simulink model "Model_FC_v14_Edit_for_Full_Scale_Fuel_Cell_GAS"  (R2017a)
settings: Solver=VariableStepAuto  StartTime=0  StopTime=10  FixedStep=0.01  MaxStep=1e-4  RelTol=1e-3  EnableMultiTasking=on
undefined symbols (not defined in the file): sigbuilder_block
libraries: powerlib x9, simulink x7, fl_lib x5, nesl_utility x3, powerlib_meascontrol x1
(part 1 of 3)
settings Model: SimulationMode=accelerator  Creator=Mina  LastModifiedBy=Mina
settings DataIOCC: LimitDataPoints=on  SaveFormat=Array
settings OptimizationCC: BlockReduction=off  ConditionallyExecuteInputs=off  LifeSpan=inf  SimCompilerOptimization=on  AccelVerboseBuild=on
settings DebuggingCC: SFUnexpectedBacktrackingDiag=warning  SFNoUnconditionalDefaultTransitionDiag=warning  SFExecutionAtInitializationDiag=none
settings HardwareCC: ProdBitPerPointer=32  ProdBitPerSizeT=32  ProdBitPerPtrDiffT=32  ProdLargestAtomicFloat=None  ProdIntDivRoundTo=Undefined  ProdEndianess=Unspecified  ProdWordSize=32  ProdHWDeviceType=32-bit Generic
settings ModelReferenceCC: PropagateSignalLabelsOutOfModel=off
settings GRTTargetCC: TargetLangStandard=C89/C90 (ANSI)  GeneratePreprocessorConditionals=Disable all
settings ConfigComp: CovMetricSettings=dw  CovHtmlReporting=on  CovSaveCumulativeToWorkspaceVar=on  CovSaveSingleToWorkspaceVar=on  CovExternalEMLEnable=off

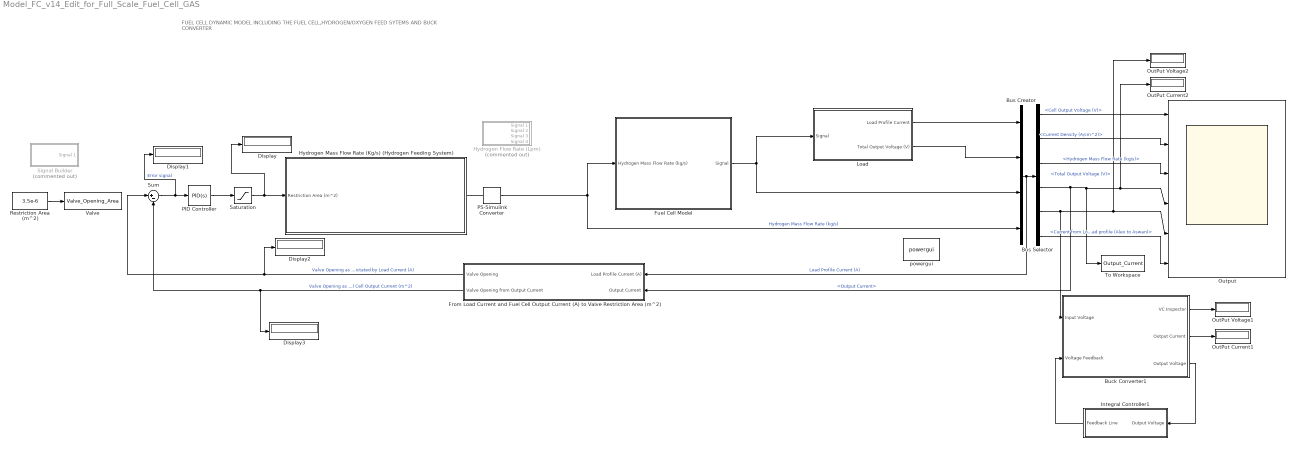
== system Model_FC_v14_Edit_for_Full_Scale_Fuel_Cell_GAS ==
  note: FUEL CELL DYNAMIC MODEL INCLUDING THE FUEL CELL,HYDROGEN/OXYGEN FEED SYTEMS AND BUCK CONVERTER
  Buck Converter1 : Subsystem
  Bus Creator : BusCreator  Inputs=4
  Bus Selector : BusSelector  OutputSignals=signal3.Cell Output Voltage (V),signal3.Current Density (A/cm^2),Hydrogen Mass Flow Rate (kg/s),signal3.Output Current,Total Output Voltage (V),Current from Load profile (Alex to Aswan)
  Display{,1..3} (4 alike) : Display
      Display settings: Decimation=100
  From Load Current and Fuel Cell Output Current (A) to Valve Restriction Area (m^2) : Subsystem
  Fuel Cell Model : Subsystem  mask(Fuel Cell Model){Temperature_c=80, Hydrogen_Pressure_atm=8, Air_Pressure_atm=8, Number_of_cells=235, Cell_Area_cm_squared=43.9714, Alpha_charge_Transfer_Coefficient=0.5, Exchange_Current_Density_i0=0.00000012246, Internal_Resistance_r=0.019, Amplification_Constant_Alpha1=0.085, Limiting_Current_Density_i_l=2, Mass_Transport_Limit_k=1.1, Dynamic_Response=[5 1]}
      mask prompts: Temperature_c "Temperature (c)"; Hydrogen_Pressure_atm "Hydrogen Pressure (atm)"; Air_Pressure_atm "Air Pressure (atm)"; Number_of_cells "Number Of Cells"; Cell_Area_cm_squared "Cell Area (cm^2)"; Alpha_charge_Transfer_Coefficient "Alpha (Charge Transfer Coefficient)"; Exchange_Current_Density_i0 "Exchange Current Density (i_0)(A/cm^2)"; Internal_Resistance_r "Internal Resistance (r)(Ohm)"; Amplification_Constant_Alpha1 "Amplification Constant (Alpha1)"; Limiting_Current_Density_i_l "Limiting Current Density (i_L)(A/cm^2)"; Mass_Transport_Limit_k "Mass Transport Limit (k)"; Dynamic_Response "Cell Dynamic Response (s)"
      mask help:
      | This is a mathematical Fuel Cell dynamic model. It operates under the Following Assumptions:
      | 1-The model is dynamic ,ie, it models the fuel cell behavior with respect to time.
      | 2-Fuel Cell Temperature is Constant.
      | 3-No Excess Hydrogen ,ie, Every Hydrogen molecule that enters the fuel cell Stack reacts to produce electricity.
      | 4-No excess Air.
      | 5-Concentration Losses are not calculated in the Model as we will never approach this region during operation.
      mask TypeOptions Temperature_c:
      | Stack Temperature
      | (C)/Value
      mask TypeOptions Hydrogen_Pressure_atm: Hydrogen Pressure (atm)/Value
      mask TypeOptions Air_Pressure_atm: Air Pressue (atm)/Value
      mask TypeOptions Number_of_cells: Number of Cells/Value
      mask TypeOptions Cell_Area_cm_squared:
      | Cell Area
      | (cm^2)/Value
      mask TypeOptions Alpha_charge_Transfer_Coefficient:
      | From Current Density (A//cm^2)
      | To
      | Overvoltages (V)/Activation Overvoltage/Alpha
      | Charge Transfer Coefficient1/Value
      mask TypeOptions Exchange_Current_Density_i0:
      | From Current Density (A//cm^2)
      | To
      | Overvoltages (V)/Activation Overvoltage/Reference Exchange Current Density
      | (I_0)1/Value
      mask TypeOptions Internal_Resistance_r:
      | From Current Density (A//cm^2)
      | To
      | Overvoltages (V)/Ohmic Overvoltage/Internal Resistance
      | (r)/Value
      mask TypeOptions Amplification_Constant_Alpha1:
      | From Current Density (A//cm^2)
      | To
      | Overvoltages (V)/Concentration Overvoltage/Amplification Constant
      | Alpha2/Value
      mask TypeOptions Limiting_Current_Density_i_l:
      | From Current Density (A//cm^2)
      | To
      | Overvoltages (V)/Concentration Overvoltage/Limiting Current
      | (i_L)1/Value
      mask TypeOptions Mass_Transport_Limit_k:
      | From Current Density (A//cm^2)
      | To
      | Overvoltages (V)/Concentration Overvoltage/Mass Transport Constant
      | (K)1/Value
      mask TypeOptions Dynamic_Response: Cell dynamic/Denominator
      mask Display: image(imread('power_fuelcell.png'));port_label('output',1,'m');
  Hydrogen Flow Rate (Lpm) : Subsystem  Tag=STV Subsys  Commented=on  LoadFcn=sigbuilder_block('load');  StartFcn=sigbuilder_block('start');  StopFcn=sigbuilder_block('stop');  ClipboardFcn=sigbuilder_block('clipboard');  mask(Sigbuilder block){tuvar=[0:10]}
      mask help: Simulink:masks:SigbuilderBlock_MD
      mask init:
      | if ~strcmp(get_param(bdroot(gcbh),'SimulationStatus'),'stopped') tuvar = sigbuilder_block('maskInit'); end
      settings: CopyFcn=sigbuilder_block('copy');  DeleteFcn=sigbuilder_block('delete');  ModelCloseFcn=sigbuilder_block('modelClose');  PreSaveFcn=sigbuilder_block('preSave');  PauseFcn=sigbuilder_block('pause');  ContinueFcn=sigbuilder_block('continue');  NameChangeFcn=sigbuilder_block('namechange');  OpenFcn=sigbuilder_block('open',[437.6 199.2 550.4 400 ]);  CloseFcn=sigbuilder_block('close');
      mask Display: plot(0, 0, 100, 100,[2, 2, 32, 32, 2], [68, 8, 8, 68, 68],[32, 2], [38, 38], [32, 19, 2],[53, 60, 44], [32, 17, 17, 2],[16, 16, 31, 31]);txt = getActiveGroup(gcbh);text(2, 100, txt,'verticalAlignment', 'top');
  Hydrogen Mass Flow Rate (Kg/s) (Hydrogen Feeding System) : Subsystem
  Integral Controller1 : Subsystem
  Load : Subsystem
  OutPut Current1 : Display
  OutPut Current2 : Display
  OutPut Voltage1 : Display
  OutPut Voltage2 : Display
  "Output " : Scope  NumInputPorts=6
  PID Controller : simulink/Continuous/PID Controller  Controller=PID  TimeDomain=Continuous-time  SampleTime=-1  IntegratorMethod=Forward Euler  FilterMethod=Forward Euler  Form=Parallel  UseFilter=on  ControllerParametersSource=internal  P=0.5  I=0.7  D=0.01  N=100  InitialConditionSource=internal  InitialConditionForIntegrator=0  InitialConditionForFilter=0  ExternalReset=none  LimitOutput=on  UpperSaturationLimit=1.5e-5  LowerSaturationLimit=-inf  LinearizeAsGain=on  AntiWindupMode=none  Kb=1  TrackingMode=off  Kt=1  PParamMin=[]  PParamMax=[]  IParamMin=[]  IParamMax=[]  DParamMin=[]  DParamMax=[]  NParamMin=[]  NParamMax=[]  KbParamMin=[]  KbParamMax=[]  KtParamMin=[]  KtParamMax=[]  POutMin=[]  POutMax=[]  IOutMin=[]  IOutMax=[]  DOutMin=[]  DOutMax=[]  NOutMin=[]  NOutMax=[]  KbOutMin=[]  KbOutMax=[]  KtOutMin=[]  KtOutMax=[]  IntegratorOutMin=[]  IntegratorOutMax=[]  FilterOutMin=[]  FilterOutMax=[]  SumOutMin=[]  SumOutMax=[]  SumI1OutMin=[]  SumI1OutMax=[]  SumI2OutMin=[]  SumI2OutMax=[]  SumI3OutMin=[]  SumI3OutMax=[]  SumDOutMin=[]  SumDOutMax=[]  SaturationOutMin=[]  SaturationOutMax=[]  IntegratorContinuousStateAttributes=''  IntegratorStateMustResolveToSignalObject=off  IntegratorRTWStateStorageClass=Auto  FilterContinuousStateAttributes=''  FilterStateMustResolveToSignalObject=off  FilterRTWStateStorageClass=Auto  DifferentiatorICPrevScaledInput=0  DifferentiatorOutMin=[]  DifferentiatorOutMax=[]  InitialConditionSetting=State (most efficient)
  PS-Simulink Converter : nesl_utility/PS-Simulink Converter  PhysicalDomain=network_engine_domain  SubClassName=ps_output  LeftPortType=input  RightPortType=output  PseudoPeriodic=off  Frequencies=[]  Unit=1  AffineConversion=off
  "Restriction Area (m^2) " : Constant  Value=3.5e-6  VectorParams1D=off
  Saturation : Saturate  UpperLimit=2.7e-5  LowerLimit=0
  Signal Builder : Subsystem  Tag=STV Subsys  Commented=on  LoadFcn=sigbuilder_block('load');  StartFcn=sigbuilder_block('start');  StopFcn=sigbuilder_block('stop');  ClipboardFcn=sigbuilder_block('clipboard');  mask(Sigbuilder block){tuvar=[0:10]}
      mask help: Simulink:masks:SigbuilderBlock_MD
      mask init:
      | if ~strcmp(get_param(bdroot(gcbh),'SimulationStatus'),'stopped') tuvar = sigbuilder_block('maskInit'); end
      settings: CopyFcn=sigbuilder_block('copy');  DeleteFcn=sigbuilder_block('delete');  ModelCloseFcn=sigbuilder_block('modelClose');  PreSaveFcn=sigbuilder_block('preSave');  PauseFcn=sigbuilder_block('pause');  ContinueFcn=sigbuilder_block('continue');  NameChangeFcn=sigbuilder_block('namechange');  OpenFcn=sigbuilder_block('open',[403.5 117 550.5 359.25 ]);  CloseFcn=sigbuilder_block('close');
      mask Display: plot(0, 0, 100, 100,[2, 2, 32, 32, 2], [68, 8, 8, 68, 68],[32, 2], [38, 38], [32, 19, 2],[53, 60, 44], [32, 17, 17, 2],[16, 16, 31, 31]);txt = getActiveGroup(gcbh);text(2, 100, txt,'verticalAlignment', 'top');
  Sum : Sum  Inputs=|+-
  To Workspace : ToWorkspace  VariableName=Output_Current  SaveFormat=Timeseries  SampleTime=-1
  Valve : ToWorkspace  VariableName=Valve_Opening_Area  SaveFormat=Timeseries  SampleTime=-1
  powergui : powerlib/powergui  Priority=1  SimulationMode=Continuous  SampleTime=50e-6  frequency=60  Iterations=50  frequencyindice=0  Pbase=100e6  ErrMax=1e-4  UnitsV=kV  UnitsW=MW  buscounter=0  FunctionMessages=off  echomessages=off  EnableUseOfTLC=off  CurrentSourceSwitches=off  DisableSnubberDevices=off  DisableRonSwitches=off  DisableVfSwitches=off  DisplayEquations=off  SolverType=Tustin/Backward Euler (TBE)  Interpol=off  ExternalGateDelay=off  methode=off  Ts=100  x0status=blocks  SPID=on  SwTol=0  HookPort=off  RestoreLinks=warning  ResistiveCurrentMeasurement=off  Frange=[0:2:500]  Ylog=off  Xlog=on  ShowGrid=off  save=off  variable=ZData  structure=0  ZoomFFT=off  StartTime=0.0  cycles=1  DisplayStyle=1  fundamental=60  FreqAxis=off  MaxFrequency=1000  frequencyindicesteady=1  RmsSteady=1  display=off
  wires:
  Fuel Cell Model/1(Signal) -> Bus Creator/3, Load/1(Signal)
  PS-Simulink Converter/1 -> Fuel Cell Model/1(Hydrogen Mass Flow Rate (kg/s)), Bus Creator/4  "Hydrogen Mass Flow Rate (kg/s)"
  Load/1(Load Profile Current) -> Bus Creator/1
  Load/2(Total Output Voltage (V)) -> Bus Creator/2
  Bus Selector/1 -> "Output "/1  "<Cell Output Voltage (V)>"
  Bus Selector/2 -> "Output "/2  "<Current Density (A/cm^2)>"
  Bus Selector/3 -> "Output "/3  "<Hydrogen Mass Flow Rate (kg/s)>"
  Bus Selector/4 -> From Load Current and Fuel Cell Output Current (A) to Valve Restriction Area (m^2)/2(Output Current), To Workspace/1, "Output "/4, OutPut Current2/1  "<Output Current>"
  Bus Selector/5 -> Buck Converter1/1(Input Voltage), OutPut Voltage2/1, "Output "/5  "<Total Output Voltage (V)>"
  Buck Converter1/1(VC Inspector) -> OutPut Voltage1/1
  Buck Converter1/3(Output Voltage) -> Integral Controller1/1(Output Voltage)
  Integral Controller1/1(Feedback Line) -> Buck Converter1/2(Voltage Feedback)
  Buck Converter1/2(Output Current) -> OutPut Current1/1
  From Load Current and Fuel Cell Output Current (A) to Valve Restriction Area (m^2)/1(Valve Opening) -> Sum/1, Display2/1  "Valve Opening as dictated by Load Current (A)"
  "Restriction Area (m^2) "/1 -> Valve/1
  From Load Current and Fuel Cell Output Current (A) to Valve Restriction Area (m^2)/2(Valve Opening from Output Current) -> Sum/2, Display3/1  "Valve Opening as dictated by Fuel Cell Output Current (m^2)"
  Sum/1 -> PID Controller/1, Display1/1  "Error signal"
  Bus Creator/1 -> From Load Current and Fuel Cell Output Current (A) to Valve Restriction Area (m^2)/1(Load Profile Current (A)), Bus Selector/1  "Load Profile Current (A)"
  Bus Selector/6 -> "Output "/6  "<Current from Load profile (Alex to Aswan)>"
  PID Controller/1 -> Saturation/1
  Saturation/1 -> Hydrogen Mass Flow Rate (Kg/s) (Hydrogen Feeding System)/1(Restriction Area (m^2)), Display/1
  connections:
  PS-Simulink Converter/LConn1 -- Hydrogen Mass Flow Rate (Kg/s) (Hydrogen Feeding System)/RConn1

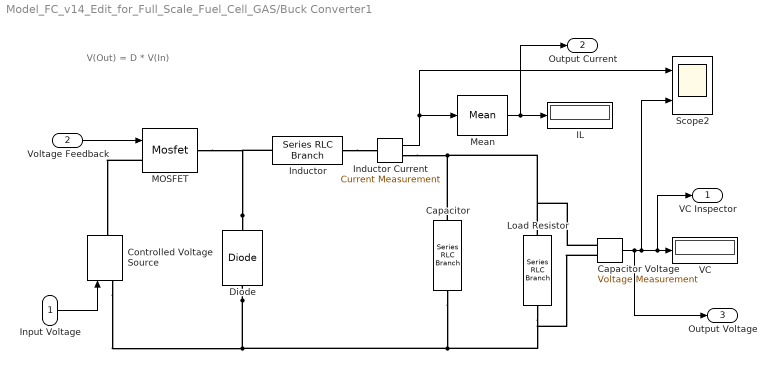
== system Model_FC_v14_Edit_for_Full_Scale_Fuel_Cell_GAS/Buck Converter1 ==
  note: V(Out) = D * V(In)
  Input Voltage : Inport
  Voltage Feedback : Inport  Port=2
  Capacitor : powerlib/Elements/Series RLC Branch  LConnTagsString=__new0  RConnTagsString=__new0  BranchType=C  Resistance=1  Inductance=1e-3  SetiL0=off  InitialCurrent=0  Capacitance=250e-6  Setx0=off  InitialVoltage=0  Measurements=None
  Capacitor Voltage : powerlib/Measurements/Voltage Measurement  PhasorSimulation=off  OutputType=Complex  PSBequivalent=0
  Controlled Voltage Source : powerlib/Electrical Sources/Controlled Voltage Source  Initialize=on  Source_Type=AC  Amplitude=0  Phase=0  Frequency=0  Measurements=None
  Diode : powerlib/Power Electronics/Diode  Ron=0.001  Lon=0  Vf=0.8  IC=0  UseSnubber=off  Rs=0  Cs=0  Measurements=off
  IL : Display
  Inductor : powerlib/Elements/Series RLC Branch  LConnTagsString=__new0  RConnTagsString=__new0  BranchType=L  Resistance=1  Inductance=1.5e-3  SetiL0=off  InitialCurrent=0  Capacitance=1e-6  Setx0=off  InitialVoltage=0  Measurements=None
  Inductor Current : powerlib/Measurements/Current Measurement  PhasorSimulation=off  OutputType=Complex  PSBequivalent=0
  Load Resistor : powerlib/Elements/Series RLC Branch  LConnTagsString=__new0  RConnTagsString=__new0  BranchType=R  Resistance=2.8  Inductance=1e-3  SetiL0=off  InitialCurrent=0  Capacitance=1e-6  Setx0=off  InitialVoltage=0  Measurements=None
  MOSFET : powerlib/Power Electronics/Mosfet  Ron=0.1  Lon=0  Rd=0.01  Vfd=0  IC=0  Rs=1e5  Cs=inf  Measurements=off
  Mean : powerlib_meascontrol/Measurements/Mean  Freq=5e3  Vinit=0  Ts=0
  Scope2 : Scope  NumInputPorts=2
  VC : Display
  VC Inspector : Outport
  Output Current : Outport  Port=2
  Output Voltage : Outport  Port=3
  wires:
  Mean/1 -> Output Current/1, IL/1
  Inductor Current/1 -> Scope2/1, Mean/1
  Voltage Feedback/1 -> MOSFET/1
  Input Voltage/1 -> Controlled Voltage Source/1
  Capacitor Voltage/1 -> Output Voltage/1, Scope2/2, VC Inspector/1, VC/1
  connections:
  Diode/RConn1 -- MOSFET/RConn1 -- Inductor/LConn1
  Inductor/RConn1 -- Inductor Current/LConn1
  Diode/LConn1 -- Controlled Voltage Source/LConn1 -- Capacitor/RConn1 -- Capacitor Voltage/LConn2 -- Load Resistor/RConn1
  Capacitor/LConn1 -- Inductor Current/RConn1 -- Load Resistor/LConn1 -- Capacitor Voltage/LConn1
  MOSFET/LConn1 -- Controlled Voltage Source/RConn1

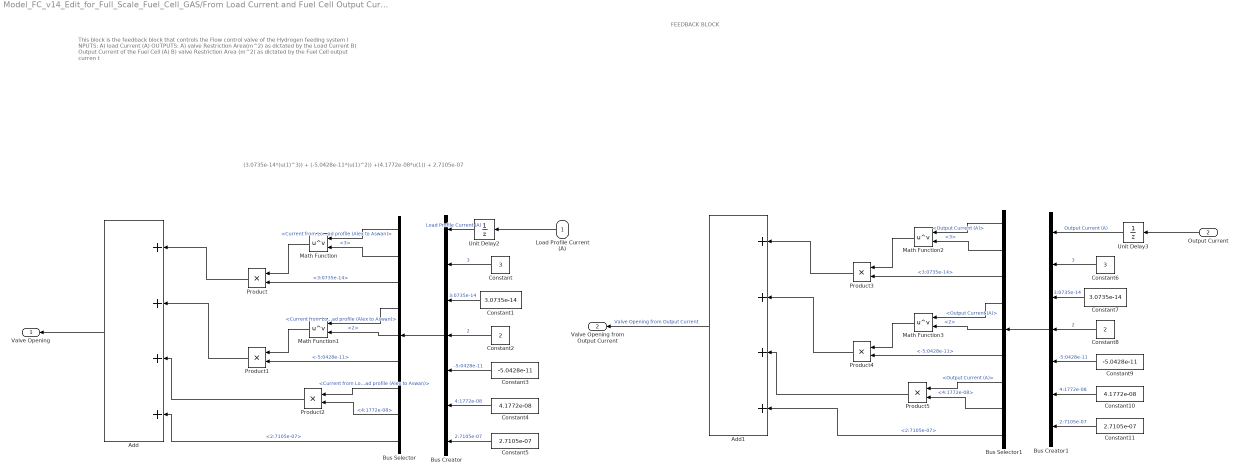
== system Model_FC_v14_Edit_for_Full_Scale_Fuel_Cell_GAS/From Load Current and Fuel Cell Output Current (A) to Valve Restriction Area (m^2) ==
  note: (3.0735e-14*(u(1)^3)) + (-5.0428e-11*(u(1)^2)) +(4.1772e-08*u(1)) + 2.7105e-07
  note: FEEDBACK BLOCK
  note: This block is the feedback block that controls the Flow control valve of the Hydrogen feeding system
      | I NPUTS: A) load Current (A) OUTPUTS: A) valve Restriction Area(m^2) as dictated by the Load Current
      | B) Output Current of the Fuel Cell (A) B) valve Restriction Area (m^2) as dictated by the Fuel Cell output curren t
  Load Profile Current (A) : Inport
  Output Current : Inport  Port=2
  Add : Sum  Inputs=4
  Add1 : Sum  Inputs=4
  Bus Creator : BusCreator  Inputs=7
  Bus Creator1 : BusCreator  Inputs=7
  Bus Selector : BusSelector  OutputSignals=Load Profile Current (A).Current from Load profile (Alex to Aswan),3,3:0735e-14,Load Profile Current (A).Current from Load profile (Alex to Aswan),2,-5:0428e-11,Load Profile Current (A).Current from Load profile (Alex to Aswan),4:1772e-08,2:7105e-07
  Bus Selector1 : BusSelector  OutputSignals=Output Current (A),3,3:0735e-14,Output Current (A),2,-5:0428e-11,Output Current (A),4:1772e-08,2:7105e-07
  Constant : Constant  Value=3
  Constant1 : Constant  Value=3.0735e-14
  Constant10 : Constant  Value=4.1772e-08
  Constant11 : Constant  Value=2.7105e-07
  Constant2 : Constant  Value=2
  Constant3 : Constant  Value=-5.0428e-11
  Constant4 : Constant  Value=4.1772e-08
  Constant5 : Constant  Value=2.7105e-07
  Constant6 : Constant  Value=3
  Constant7 : Constant  Value=3.0735e-14
  Constant8 : Constant  Value=2
  Constant9 : Constant  Value=-5.0428e-11
  Math Function{,1..3} (4 alike) : Math  Operator=pow  SaturateOnIntegerOverflow=on
  Product{,1..5} (6 alike) : Product
  Unit Delay2 : UnitDelay  SampleTime=-1
  Unit Delay3 : UnitDelay  SampleTime=-1
  Valve Opening : Outport
  Valve Opening from Output Current : Outport  Port=2
  wires:
  Load Profile Current (A)/1 -> Unit Delay2/1
  Unit Delay2/1 -> Bus Creator/1  "Load Profile Current (A)"
  Constant/1 -> Bus Creator/2  "3"
  Constant1/1 -> Bus Creator/3  "3:0735e-14"
  Constant2/1 -> Bus Creator/4  "2"
  Constant3/1 -> Bus Creator/5  "-5:0428e-11"
  Constant4/1 -> Bus Creator/6  "4:1772e-08"
  Constant5/1 -> Bus Creator/7  "2:7105e-07"
  Bus Creator/1 -> Bus Selector/1
  Bus Selector/1 -> Math Function/1  "<Current from Load profile (Alex to Aswan)>"
  Bus Selector/2 -> Math Function/2  "<3>"
  Math Function/1 -> Product/1
  Bus Selector/3 -> Product/2  "<3:0735e-14>"
  Product/1 -> Add/1
  Bus Selector/4 -> Math Function1/1  "<Current from Load profile (Alex to Aswan)>"
  Bus Selector/5 -> Math Function1/2  "<2>"
  Math Function1/1 -> Product1/1
  Bus Selector/6 -> Product1/2  "<-5:0428e-11>"
  Product1/1 -> Add/2
  Bus Selector/7 -> Product2/1  "<Current from Load profile (Alex to Aswan)>"
  Bus Selector/8 -> Product2/2  "<4:1772e-08>"
  Product2/1 -> Add/3
  Bus Selector/9 -> Add/4  "<2:7105e-07>"
  Add/1 -> Valve Opening/1
  Add1/1 -> Valve Opening from Output Current/1  "Valve Opening from Output Current"
  Constant11/1 -> Bus Creator1/7  "2:7105e-07"
  Bus Selector1/9 -> Add1/4  "<2:7105e-07>"
  Bus Selector1/5 -> Math Function3/2  "<2>"
  Constant10/1 -> Bus Creator1/6  "4:1772e-08"
  Bus Selector1/2 -> Math Function2/2  "<3>"
  Bus Creator1/1 -> Bus Selector1/1
  Constant6/1 -> Bus Creator1/2  "3"
  Constant9/1 -> Bus Creator1/5  "-5:0428e-11"
  Bus Selector1/6 -> Product4/2  "<-5:0428e-11>"
  Bus Selector1/8 -> Product5/2  "<4:1772e-08>"
  Bus Selector1/3 -> Product3/2  "<3:0735e-14>"
  Bus Selector1/7 -> Product5/1  "<Output Current (A)>"
  Constant7/1 -> Bus Creator1/3  "3:0735e-14"
  Product3/1 -> Add1/1
  Math Function2/1 -> Product3/1
  Math Function3/1 -> Product4/1
  Bus Selector1/4 -> Math Function3/1  "<Output Current (A)>"
  Product4/1 -> Add1/2
  Product5/1 -> Add1/3
  Constant8/1 -> Bus Creator1/4  "2"
  Output Current/1 -> Unit Delay3/1
  Unit Delay3/1 -> Bus Creator1/1  "Output Current (A)"
  Bus Selector1/1 -> Math Function2/1  "<Output Current (A)>"

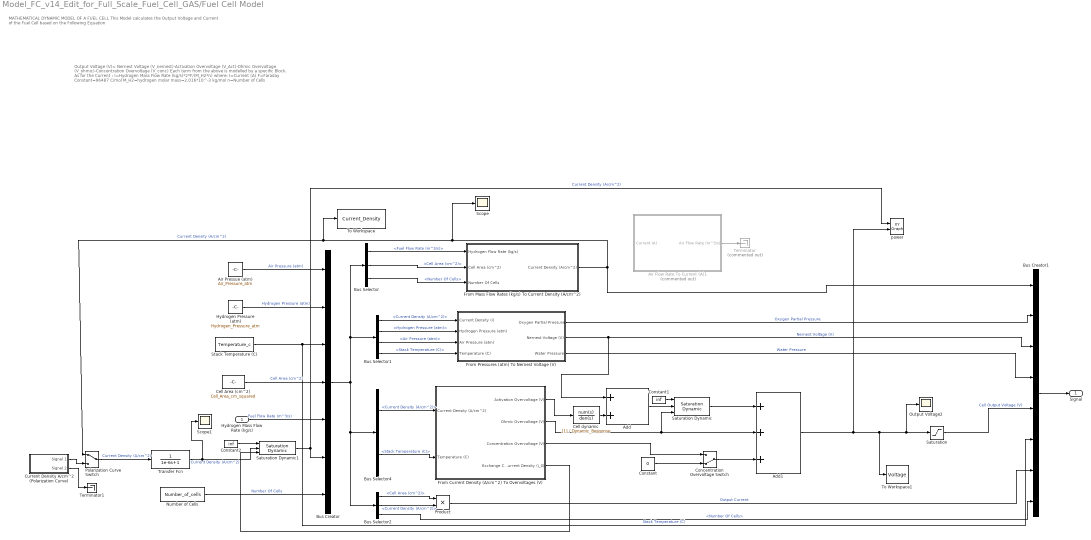
== system Model_FC_v14_Edit_for_Full_Scale_Fuel_Cell_GAS/Fuel Cell Model ==
  note: Output Voltage (V)= Nernest Voltage (V_nernest)-Activation Overvoltage (V_Act)-Ohmic Overvoltage (V_ohmic)-Concentration Overvoltage (V_conc)
      | Each term from the above is modelled by a specific Block.
      | As for the Current :
      |
      | I=Hydrogen Mass Flow Rate (kg/s)*2*F/(M_H2*n)
      | where: I=Current (A)
      | F=Faraday Constant=96487 C/mol
      | M_H2=hydrogen molar mass=2.016*10^-3 kg/mol
      | n=Number of Cells
  note: MATHEMATICAL DYNAMIC MODEL OF A FUEL CELL
      | This Model calculates the Output Voltage and Current of the Fuel Cell based on the Following Equation
  Hydrogen Mass Flow Rate (kg/s) : Inport
  " From Current Density (A/cm^2) To Overvoltages (V)" : Subsystem
  Add : Sum
  Add1 : Sum  Inputs=+++
  Air Flow Rate To Current (A)1 : Subsystem  Commented=on
  Air Pressue (atm) : Constant  Value=Air_Pressure_atm
  Bus Creator : BusCreator  Inputs=7
  Bus Creator1 : BusCreator  Inputs=8
  Bus Selector : BusSelector  OutputSignals=Fuel Flow Rate (m^3/s),Cell Area (cm^2),Number Of Cells
  Bus Selector1 : BusSelector  OutputSignals=Current Density (A/cm^2),Hydrogen Pressure (atm),Air Pressure (atm),Stack Temperature (C)
  Bus Selector2 : BusSelector  OutputSignals=Cell Area (cm^2),Current Density (A/cm^2),Number Of Cells
  Bus Selector4 : BusSelector  OutputSignals=Current Density (A/cm^2),Stack Temperature (C)
  Cell Area (cm^2) : Constant  Value=Cell_Area_cm_squared
  Cell dynamic : TransferFcn  Denominator=Dynamic_Response
  Concentration Overvoltage Switch : ManualSwitch  CurrentSetting=0
  Constant : Constant  Value=0
  Constant1 : Constant  Value=inf
  Constant2 : Constant  Value=inf
  Current Density A/cm^2 (Polarization Curve) : Subsystem  Tag=STV Subsys  LoadFcn=sigbuilder_block('load');  StartFcn=sigbuilder_block('start');  StopFcn=sigbuilder_block('stop');  ClipboardFcn=sigbuilder_block('clipboard');  mask(Sigbuilder block){tuvar=[0:10]}
      mask help: Simulink:masks:SigbuilderBlock_MD
      mask init:
      | if ~strcmp(get_param(bdroot(gcbh),'SimulationStatus'),'stopped') tuvar = sigbuilder_block('maskInit'); end
      settings: CopyFcn=sigbuilder_block('copy');  DeleteFcn=sigbuilder_block('delete');  ModelCloseFcn=sigbuilder_block('modelClose');  PreSaveFcn=sigbuilder_block('preSave');  PauseFcn=sigbuilder_block('pause');  ContinueFcn=sigbuilder_block('continue');  NameChangeFcn=sigbuilder_block('namechange');  OpenFcn=sigbuilder_block('open',[403.5 117 550.5 359.25 ]);  CloseFcn=sigbuilder_block('close');
      mask Display: plot(0, 0, 100, 100,[2, 2, 32, 32, 2], [68, 8, 8, 68, 68],[32, 2], [38, 38], [32, 19, 2],[53, 60, 44], [32, 17, 17, 2],[16, 16, 31, 31]);txt = getActiveGroup(gcbh);text(2, 100, txt,'verticalAlignment', 'top');
  From Mass Flow Rates (kg/s) To Current Density (A/cm^2) : Subsystem
  From Pressures (atm) To Nernest Voltage (V) : Subsystem
  Hydrogen Pressure (atm) : Constant  Value=Hydrogen_Pressure_atm
  Number of Cells : Constant  Value=Number_of_cells
  Output Voltage2 : Scope
  Polarization Curve Switch : ManualSwitch
  Product : Product
  Saturation : Saturate  UpperLimit=inf  LowerLimit=0  ZeroCross=off
  Saturation Dynamic : simulink/Discontinuities/Saturation Dynamic  OutMin=[]  OutMax=[]  OutDataTypeStr=Inherit: Same as second input  OutDataType=sfix(16)  OutScaling=2^-10  DoSatur=off
  Saturation Dynamic1 : simulink/Discontinuities/Saturation Dynamic  OutMin=[]  OutMax=[]  OutDataTypeStr=Inherit: Same as second input  OutDataType=sfix(16)  OutScaling=2^-10  DoSatur=off
  Scope : Scope
  Scope1 : Scope
  Stack Temperature (C) : Constant  Value=Temperature_c
  Terminator : Terminator  Commented=on
  Terminator1 : Terminator
  To Workspace : ToWorkspace  VariableName=Current_Density  SampleTime=-1
      settings: Save2DSignal=2-D array (concatenate along first dimension)
  To Workspace1 : ToWorkspace  VariableName=Voltage  SampleTime=-1
      settings: Save2DSignal=2-D array (concatenate along first dimension)
  Transfer Fcn : TransferFcn  Denominator=[1e-6 1]
  power : simulink/Sinks/XY Graph  xmin=0  xmax=20  ymin=0.0  ymax=20  st=0
  Signal : Outport
  wires:
  Saturation/1 -> Bus Creator1/5  "Cell Output Voltage (V)"
  Current Density A/cm^2 (Polarization Curve)/1(Signal 1) -> Polarization Curve Switch/2
  Hydrogen Mass Flow Rate (kg/s)/1 -> Bus Creator/5  "Fuel Flow Rate (m^3/s)"
  Bus Creator/1 -> Bus Selector2/1, Bus Selector4/1, Bus Selector1/1, Bus Selector/1
  From Mass Flow Rates (kg/s) To Current Density (A/cm^2)/1(Current Density (A/cm^2)) -> Bus Creator1/1, Scope/1, To Workspace/1, Polarization Curve Switch/1  "Current Density (A/cm^2)"
  Bus Selector/1 -> From Mass Flow Rates (kg/s) To Current Density (A/cm^2)/1(Hydrogen Flow Rate (kg/s))  "<Fuel Flow Rate (m^3/s)>"
  Bus Selector/2 -> From Mass Flow Rates (kg/s) To Current Density (A/cm^2)/2(Cell Area (cm^2))  "<Cell Area (cm^2)>"
  From Pressures (atm) To Nernest Voltage (V)/2(Nernest Voltage (V)) -> Bus Creator1/3, Add/1  "Nernest Voltage (V)"
  Bus Selector1/1 -> From Pressures (atm) To Nernest Voltage (V)/1(Current Density (i))  "<Current Density (A/cm^2)>"
  Bus Selector1/2 -> From Pressures (atm) To Nernest Voltage (V)/2(Hydrogen Pressure (atm))  "<Hydrogen Pressure (atm)>"
  Bus Selector1/3 -> From Pressures (atm) To Nernest Voltage (V)/3(Air Pressure (atm))  "<Air Pressure (atm)>"
  Bus Selector1/4 -> From Pressures (atm) To Nernest Voltage (V)/4(Temperature (C))  "<Stack Temperature (C)>"
  From Pressures (atm) To Nernest Voltage (V)/1(Oxygen Partial Pressure) -> Bus Creator1/2  "Oxygen Partial Pressure"
  From Pressures (atm) To Nernest Voltage (V)/3(Water Pressure) -> Bus Creator1/4  "Water Pressure"
  Bus Selector4/1 -> " From Current Density (A/cm^2) To Overvoltages (V)"/1(Current Density (A/cm^2))  "<Current Density (A/cm^2)>"
  Bus Selector4/2 -> " From Current Density (A/cm^2) To Overvoltages (V)"/2(Temperature (C))  "<Stack Temperature (C)>"
  " From Current Density (A/cm^2) To Overvoltages (V)"/1(Activation Overvoltage (V)) -> Cell dynamic/1
  Bus Creator1/1 -> Signal/1
  Polarization Curve Switch/1 -> Transfer Fcn/1  "Current Density (A/cm^2)"
  Constant2/1 -> Saturation Dynamic1/1
  " From Current Density (A/cm^2) To Overvoltages (V)"/4(Exchange Current Density (i_0)) -> Saturation Dynamic1/3
  Add1/1 -> power/2, To Workspace1/1, Output Voltage2/1, Saturation/1
  Cell dynamic/1 -> Add/2
  Add/1 -> Saturation Dynamic/2
  Constant1/1 -> Saturation Dynamic/1
  Saturation Dynamic/1 -> Add1/1
  " From Current Density (A/cm^2) To Overvoltages (V)"/3(Concentration Overvoltage (V)) -> Concentration Overvoltage Switch/1
  Bus Selector2/2 -> Product/2  "<Current Density (A/cm^2)>"
  Bus Selector2/1 -> Product/1  "<Cell Area (cm^2)>"
  Product/1 -> Bus Creator1/7  "Output Current"
  Bus Selector/3 -> From Mass Flow Rates (kg/s) To Current Density (A/cm^2)/3(Number Of Cells)  "<Number Of Cells>"
  Bus Selector2/3 -> Bus Creator1/8  "<Number Of Cells>"
  Saturation Dynamic1/1 -> Bus Creator/6, power/1  "Current Density (A/cm^2)"
  Transfer Fcn/1 -> Scope1/1, Saturation Dynamic1/2  "Current Density (A/cm^2)"
  Stack Temperature (C)/1 -> Bus Creator/3, Bus Creator1/6  "Stack Temperature (C)"
  Hydrogen Pressure (atm)/1 -> Bus Creator/2  "Hydrogen Pressure (atm)"
  Air Pressue (atm)/1 -> Bus Creator/1  "Air Pressure (atm)"
  Number of Cells/1 -> Bus Creator/7  "Number Of Cells"
  Cell Area (cm^2)/1 -> Bus Creator/4  "Cell Area (cm^2)"
  " From Current Density (A/cm^2) To Overvoltages (V)"/2(Ohmic Overvoltage (V)) -> Saturation Dynamic/3, Add1/2
  Concentration Overvoltage Switch/1 -> Add1/3
  Constant/1 -> Concentration Overvoltage Switch/2
  Air Flow Rate To Current (A)1/1(Air Flow Rate (m^3/s)) -> Terminator/1
  Current Density A/cm^2 (Polarization Curve)/2(Signal 2) -> Terminator1/1

== system Model_FC_v14_Edit_for_Full_Scale_Fuel_Cell_GAS/Hydrogen Flow Rate (Lpm) ==
  Demux : Demux  Tag=STV Demux
  FromWs : FromWorkspace  Tag=STV FromWs  VariableName=tuvar  SampleTime=0
      SigBuilderData=|
      | common.afterFinalStr = 'Extrapolate'
      | common.sampleTime = 0
      | dataSet.timeRange = [0 50]
      | dataSet.name = 'Group 1'
      | sbobj.Groups.Name = 'Group 1'
      | sbobj.Groups.Signals(1).Name = 'Signal 1'
      | sbobj.Groups.Signals(1).XData = [0 5 7.5 50]
      | sbobj.Groups.Signals(1).YData = [2.5 2.5 4 4]
      | sbobj.Groups.Signals(2).Name = 'Signal 2'
      | sbobj.Groups.Signals(2).XData = [0 5 5 50]
      | sbobj.Groups.Signals(2).YData = [2.5 2.5 4 4]
      | sbobj.Groups.Signals(3).Name = 'Signal 3'
      | sbobj.Groups.Signals(3).XData = [0 5 10 50]
      | sbobj.Groups.Signals(3).YData = [50 50 85 85]
      | sbobj.Groups.Signals(4).Name = 'Signal 4'
      | sbobj.Groups.Signals(4).XData = [0 50]
      | sbobj.Groups.Signals(4).YData = [170 170]
      | sbobj.Groups.TimeRange = [0 50]
  Signal 1 : Outport  Tag=STV Outport
  Signal 2 : Outport  Tag=STV Outport  Port=2
  Signal 3 : Outport  Tag=STV Outport  Port=3
  Signal 4 : Outport  Tag=STV Outport  Port=4
  wires:
  Demux/1 -> Signal 1/1
  FromWs/1 -> Demux/1
  Demux/2 -> Signal 2/1
  Demux/3 -> Signal 3/1
  Demux/4 -> Signal 4/1
